simulink model "exp2"  (R2021b)
settings: Solver=VariableStepAuto  StartTime=0.0  StopTime=10.0  RelTol=1e-3
settings Model: Creator=ashir  LastModifiedBy=ashir

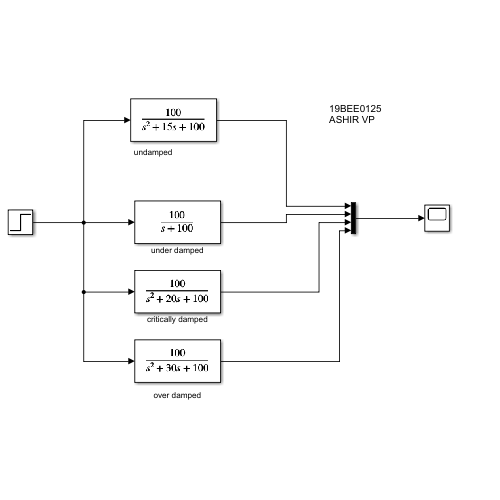
[thumbnail: Simulink's stored preview of the top-level diagram]
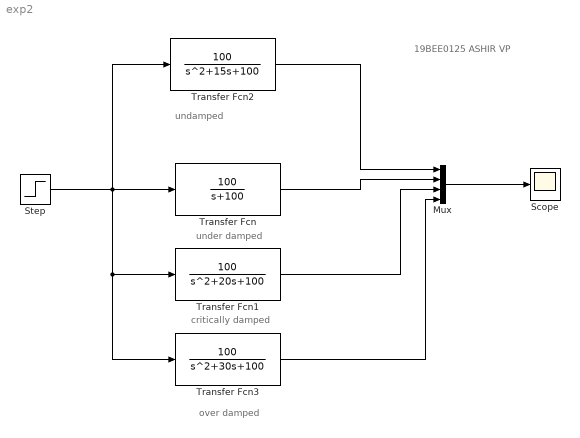
== system exp2 ==
  note: 19BEE0125
      | ASHIR VP
  note: undamped
  note: critically damped
  note: over damped
  note: under damped
  Mux : Mux
  Scope : Scope
  Step : Step  Time=0  SampleTime=0
  Transfer Fcn : TransferFcn  Numerator=[100]  Denominator=[1 100]
  Transfer Fcn1 : TransferFcn  Numerator=[100]  Denominator=[1 20 100]
  Transfer Fcn2 : TransferFcn  Numerator=[100]  Denominator=[1 15 100]
  Transfer Fcn3 : TransferFcn  Numerator=[100]  Denominator=[1 30 100]
  wires:
  Step/1 -> Transfer Fcn3/1, Transfer Fcn1/1, Transfer Fcn2/1, Transfer Fcn/1
  Transfer Fcn2/1 -> Mux/1
  Transfer Fcn/1 -> Mux/2
  Transfer Fcn1/1 -> Mux/3
  Transfer Fcn3/1 -> Mux/4
  Mux/1 -> Scope/1
